simulink model "fetft_recurrent_hybrid_write_hold_read"  (R2026a)
settings: Solver=FixedStepDiscrete  StopTime=8e-05  FixedStep=5e-08
InitFcn:
  | recurrentHybridInput = fetft_recurrent_hybrid_dataset;
settings Model: Creator=elesamj  LastModifiedBy=elesamj

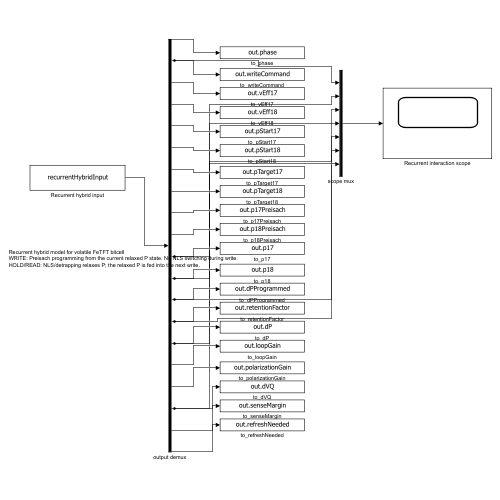
[thumbnail: Simulink's stored preview of the top-level diagram]
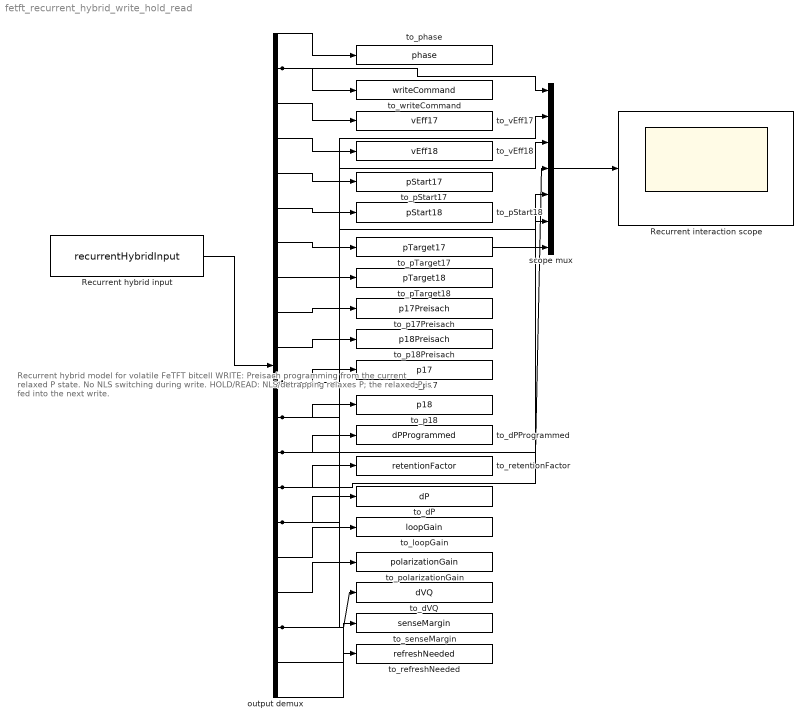
== system fetft_recurrent_hybrid_write_hold_read ==
  note: Recurrent hybrid model for volatile FeTFT bitcell
      | WRITE: Preisach programming from the current relaxed P state. No NLS switching during write.
      | HOLD/READ: NLS/detrapping relaxes P; the relaxed P is fed into the next write.
  Recurrent hybrid input : FromWorkspace  VariableName=recurrentHybridInput  Interpolate=off  OutputAfterFinalValue=Holding final value
  Recurrent interaction scope : Scope
  output demux : Demux  Outputs=20
  scope mux : Mux  Inputs=7
  to_dP : ToWorkspace  VariableName=dP  SaveFormat=Structure With Time  SampleTime=-1
  to_dPProgrammed : ToWorkspace  VariableName=dPProgrammed  SaveFormat=Structure With Time  SampleTime=-1
  to_dVQ : ToWorkspace  VariableName=dVQ  SaveFormat=Structure With Time  SampleTime=-1
  to_loopGain : ToWorkspace  VariableName=loopGain  SaveFormat=Structure With Time  SampleTime=-1
  to_p17 : ToWorkspace  VariableName=p17  SaveFormat=Structure With Time  SampleTime=-1
  to_p17Preisach : ToWorkspace  VariableName=p17Preisach  SaveFormat=Structure With Time  SampleTime=-1
  to_p18 : ToWorkspace  VariableName=p18  SaveFormat=Structure With Time  SampleTime=-1
  to_p18Preisach : ToWorkspace  VariableName=p18Preisach  SaveFormat=Structure With Time  SampleTime=-1
  to_pStart17 : ToWorkspace  VariableName=pStart17  SaveFormat=Structure With Time  SampleTime=-1
  to_pStart18 : ToWorkspace  VariableName=pStart18  SaveFormat=Structure With Time  SampleTime=-1
  to_pTarget17 : ToWorkspace  VariableName=pTarget17  SaveFormat=Structure With Time  SampleTime=-1
  to_pTarget18 : ToWorkspace  VariableName=pTarget18  SaveFormat=Structure With Time  SampleTime=-1
  to_phase : ToWorkspace  VariableName=phase  SaveFormat=Structure With Time  SampleTime=-1
  to_polarizationGain : ToWorkspace  VariableName=polarizationGain  SaveFormat=Structure With Time  SampleTime=-1
  to_refreshNeeded : ToWorkspace  VariableName=refreshNeeded  SaveFormat=Structure With Time  SampleTime=-1
  to_retentionFactor : ToWorkspace  VariableName=retentionFactor  SaveFormat=Structure With Time  SampleTime=-1
  to_senseMargin : ToWorkspace  VariableName=senseMargin  SaveFormat=Structure With Time  SampleTime=-1
  to_vEff17 : ToWorkspace  VariableName=vEff17  SaveFormat=Structure With Time  SampleTime=-1
  to_vEff18 : ToWorkspace  VariableName=vEff18  SaveFormat=Structure With Time  SampleTime=-1
  to_writeCommand : ToWorkspace  VariableName=writeCommand  SaveFormat=Structure With Time  SampleTime=-1
  wires:
  output demux/1 -> to_phase/1
  output demux/2 -> to_writeCommand/1, scope mux/1
  output demux/3 -> to_vEff17/1
  output demux/4 -> to_vEff18/1
  output demux/5 -> to_pStart17/1
  output demux/6 -> to_pStart18/1
  output demux/7 -> to_pTarget17/1
  output demux/8 -> to_pTarget18/1
  output demux/9 -> to_p17Preisach/1
  output demux/10 -> to_p18Preisach/1
  output demux/11 -> to_p17/1, scope mux/2
  output demux/12 -> to_p18/1, scope mux/3
  output demux/13 -> to_dPProgrammed/1, scope mux/4
  output demux/14 -> to_retentionFactor/1, scope mux/5
  output demux/15 -> to_dP/1, scope mux/6
  output demux/16 -> to_loopGain/1
  output demux/17 -> to_polarizationGain/1
  output demux/18 -> to_dVQ/1, scope mux/7
  output demux/19 -> to_senseMargin/1
  output demux/20 -> to_refreshNeeded/1
  Recurrent hybrid input/1 -> output demux/1
  scope mux/1 -> Recurrent interaction scope/1
